simulink model "ref4_xy"  (Simulink 4.00)
settings: Solver=FixedStepDiscrete  StartTime=0.0  StopTime=inf  FixedStep=Ts  RelTol=1e-3
values from neighbouring files (symbols this model uses):
  Ts = 5e-3    (= 0.005)    [makeplant.m]    (also in profile3.m = acc; recalc.m = 0.001)
libraries: simulink3 x3, motion x1
settings Model: LastModifiedBy=plambrec  BlockReductionOpt=off

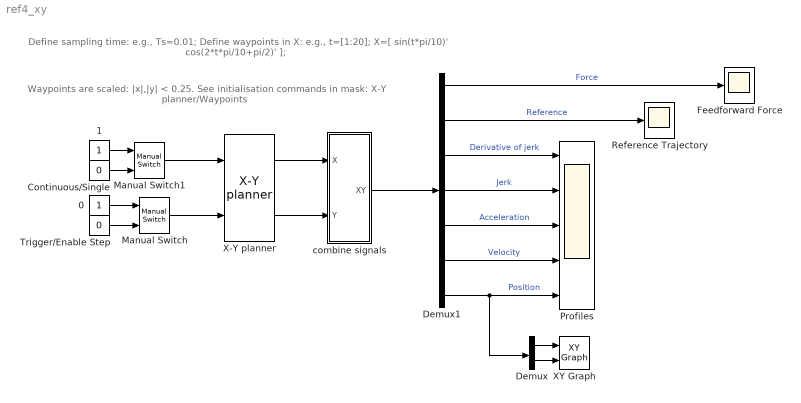
== system ref4_xy ==
  note: Define sampling time: e.g.,   Ts=0.01;
      | Define waypoints in X:  e.g.,   t=[1:20]; X=[ sin(t*pi/10)' cos(2*t*pi/10+pi/2)' ];
  note: Waypoints are scaled: |x|,|y| < 0.25.
      | See initialisation commands in mask: X-Y planner/Waypoints
  0 : Constant  Value=1
  1 : Constant  Value=1
  Continuous/Single : Constant  Value=0
  Demux : Demux  Outputs=2  BusSelectionMode=off
  Demux1 : Demux  Outputs=7  BusSelectionMode=off
  Feedforward Force : Scope
      settings: TimeRange=3  YMin=-150  YMax=175  SaveToWorkspace=off  SaveName=ScopeData  LimitDataPoints=on  MaxDataPoints=50000
  Manual Switch : simulink3/Nonlinear/Manual Switch  sw=0  action=0
  Manual Switch1 : simulink3/Nonlinear/Manual Switch  sw=1  action=0
  Profiles : Scope  NumInputPorts=5
      settings: TimeRange=25  YMin=-20000~-200~-2~-0.2~-0.4  YMax=20000~200~2~0.2~0.4  SaveToWorkspace=off  SaveName=ScopeData2  LimitDataPoints=on  MaxDataPoints=5000000
  Reference Trajectory : Scope
      settings: TimeRange=3  YMin=-0.2  YMax=1.2  SaveToWorkspace=off  LimitDataPoints=on  MaxDataPoints=50000
  Trigger/Enable Step : Constant  Value=0
  "X-Y planner " : motion/Real Time/X-Y planner   Ts=Ts  Tsettle=1  X=X
  XY Graph : simulink3/Sinks/XY Graph  xmin=-.3  xmax=.3  ymin=-.3  ymax=.3  st=-1
  "combine signals " : Subsystem
      settings: RTWFcnNameOpts=Auto  RTWFileNameOpts=Auto
  wires:
  Demux1/1 -> Feedforward Force/1  "Force"
  Demux1/2 -> Reference Trajectory/1  "Reference"
  Demux1/3 -> Profiles/1  "Derivative of jerk"
  Demux1/4 -> Profiles/2  "Jerk"
  Demux1/5 -> Profiles/3  "Acceleration"
  Demux1/6 -> Profiles/4  "Velocity"
  Demux1/7 -> Profiles/5, Demux/1  "Position"
  Trigger/Enable Step/1 -> Manual Switch/2
  0/1 -> Manual Switch/1
  "combine signals "/1(XY) -> Demux1/1
  Demux/1 -> XY Graph/1
  Demux/2 -> XY Graph/2
  Continuous/Single/1 -> Manual Switch1/2
  1/1 -> Manual Switch1/1
  "X-Y planner "/1 -> "combine signals "/1(X)
  "X-Y planner "/2 -> "combine signals "/2(Y)
  Manual Switch/1 -> "X-Y planner "/2
  Manual Switch1/1 -> "X-Y planner "/1

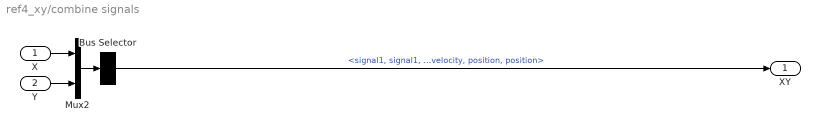
== system ref4_xy/combine signals  ==
  X : Inport  Port=1
  Y : Inport  Port=2
  Bus Selector : BusSelector  OutputSignals=signal1.signal1,signal2.signal1,signal1.signal2,signal2.signal2,signal1.signal3.derivative of jerk,signal2.signal3.derivative of jerk,signal1.signal3.jerk,signal2.signal3.jerk,signal1.signal3.acceleration,signal2.signal3.acceleration,signal1.signal3.velocity,signal2.signal3.velocity,signal1.signal3.position,signal2.signal3.position  MuxedOutput=on
  Mux2 : Mux  Inputs=2
  XY : Outport  Port=1
  wires:
  Mux2/1 -> Bus Selector/1
  X/1 -> Mux2/1
  Bus Selector/1 -> XY/1  "<signal1, signal1, signal2, signal2, derivative of jerk, derivative of jerk, jerk, jerk, acceleration, acceleration, velocity, velocity, position, position>"
  Y/1 -> Mux2/2
